simulink model "quat_compute_J2000_to_body_est"  (R2014b)
settings: Solver=FixedStepDiscrete  StartTime=0.0  StopTime=sim_time_step_size  FixedStep=sim_time_step_size  RelTol=1e-3
undefined symbols (not defined in the file or in its folder): ini_quaternion_topo_to_body_est, sim_time_step_size
libraries: util_frame_rotation_lib x2, util_quat_lib x2
settings Model: Creator=Jim Kaidy  LastModifiedBy=mstewart
settings DataIOCC: SignalLoggingSaveFormat=ModelDataLogs
settings OptimizationCC: ExpressionDepthLimit=2147483647
settings DebuggingCC: UnderspecifiedInitializationDetection=Classic  MergeDetectMultiDrivingBlocksExec=none  FcnCallInpInsideContextMsg=EnableAllAsWarning  StateNameClashWarn=warning

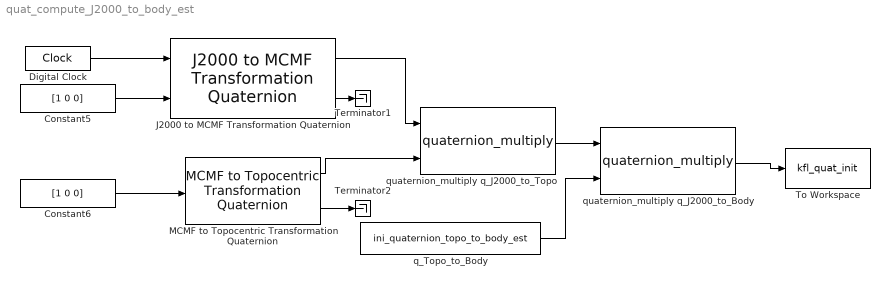
== system quat_compute_J2000_to_body_est ==
  Constant5 : Constant  Value=[1 0 0]
  Constant6 : Constant  Value=[1 0 0]
  Digital Clock : DigitalClock  SampleTime=sim_time_step_size
  J2000 to MCMF Transformation Quaternion : util_frame_rotation_lib/J2000 to MCMF  Transformation Quaternion  SystemSampleTime=-1
  MCMF to Topocentric Transformation Quaternion : util_frame_rotation_lib/MCMF to Topocentric  Transformation Quaternion  SystemSampleTime=-1
  Terminator1 : Terminator
  Terminator2 : Terminator
  To Workspace : ToWorkspace  VariableName=kfl_quat_init  SampleTime=-1
      settings: MaxDataPoints=1
  q_Topo_to_Body : Constant  Value=ini_quaternion_topo_to_body_est
  quaternion_multiply q_J2000_to_Body : util_quat_lib/quaternion_multiply  SystemSampleTime=-1
  quaternion_multiply q_J2000_to_Topo : util_quat_lib/quaternion_multiply  SystemSampleTime=-1
  wires:
  J2000 to MCMF Transformation Quaternion/2 -> Terminator1/1
  MCMF to Topocentric Transformation Quaternion/2 -> Terminator2/1
  Digital Clock/1 -> J2000 to MCMF Transformation Quaternion/1
  Constant5/1 -> J2000 to MCMF Transformation Quaternion/2
  J2000 to MCMF Transformation Quaternion/1 -> quaternion_multiply q_J2000_to_Topo/1
  MCMF to Topocentric Transformation Quaternion/1 -> quaternion_multiply q_J2000_to_Topo/2
  Constant6/1 -> MCMF to Topocentric Transformation Quaternion/1
  quaternion_multiply q_J2000_to_Topo/1 -> quaternion_multiply q_J2000_to_Body/1
  q_Topo_to_Body/1 -> quaternion_multiply q_J2000_to_Body/2
  quaternion_multiply q_J2000_to_Body/1 -> To Workspace/1
